simulink library "typhoonPatterns"  (R2019a)
settings: Solver=VariableStepAuto  StartTime=0.0  StopTime=10.0  RelTol=1e-3
undefined symbols (not defined in the file or in its folder): c_clamp, C_l, c_picoup_mat, c_picoup_seq, cc_berg, crun_sp_ind, cst_sp_ind, f, f_picoup, f_sp_ind, fc, Jm, L, L1, L2, L_l, l_picoup_mat, l_picoup_seq, l_rl, La_DC, lc_berg, Lc_sm, Ld, length_rl, Lf_DC, Llfd_sm, Llkd_sm, Llkq_sm, Llr1_ind, Llr2_ind, Llr_ind, llrm_sp_ind, Lls_ind, Lls_sm, llsa_sp_ind, llsm_sp_ind, Lm, Lmd_sm, Lmq_sm, Lq, n1, n2, nanm_sp_ind, pms, R, R1, R2, r_clamp, R_l, r_picoup_mat, r_picoup_seq, r_rl, Ra_DC, rc_berg, Rf_DC, Rf_sm, Rkd_sm, Rkq_sm, Rm, Rr1_ind ... (+10)
libraries: powerlib x281
(part 3 of 3)

== system typhoonPatterns/RL Section 4PH ==
  RL1 : powerlib/Elements/Series RLC Branch  LConnTagsString=__new0  RConnTagsString=__new0  BranchType=RL  Resistance=R  Inductance=L  SetiL0=off  InitialCurrent=0  Capacitance=1e-6  Setx0=off  InitialVoltage=0  Measurements=None
      settings: SourceProductName=Simscape Electrical
  RL2 : powerlib/Elements/Series RLC Branch  LConnTagsString=__new0  RConnTagsString=__new0  BranchType=RL  Resistance=r_rl*length_rl  Inductance=l_rl*length_rl  SetiL0=off  InitialCurrent=0  Capacitance=1e-6  Setx0=off  InitialVoltage=0  Measurements=None
      settings: SourceProductName=Simscape Electrical
  RL3 : powerlib/Elements/Series RLC Branch  LConnTagsString=__new0  RConnTagsString=__new0  BranchType=RL  Resistance=r_rl*length_rl  Inductance=l_rl*length_rl  SetiL0=off  InitialCurrent=0  Capacitance=1e-6  Setx0=off  InitialVoltage=0  Measurements=None
      settings: SourceProductName=Simscape Electrical
  RL4 : powerlib/Elements/Series RLC Branch  LConnTagsString=__new0  RConnTagsString=__new0  BranchType=RL  Resistance=r_rl*length_rl  Inductance=l_rl*length_rl  SetiL0=off  InitialCurrent=0  Capacitance=1e-6  Setx0=off  InitialVoltage=0  Measurements=None
      settings: SourceProductName=Simscape Electrical
  a_in : PMIOPort  Side=Left
  a_out : PMIOPort  Port=2  Side=Right
  b_in : PMIOPort  Port=3  Side=Left
  b_out : PMIOPort  Port=4  Side=Right
  c_in : PMIOPort  Port=5  Side=Left
  c_out : PMIOPort  Port=6  Side=Right
  d_in : PMIOPort  Port=7  Side=Left
  d_out : PMIOPort  Port=8  Side=Right
  connections:
  RL2/RConn1 -- b_out/RConn1
  a_out/RConn1 -- RL1/RConn1
  a_in/RConn1 -- RL1/LConn1
  RL2/LConn1 -- b_in/RConn1
  RL3/LConn1 -- c_in/RConn1
  RL3/RConn1 -- c_out/RConn1
  RL4/RConn1 -- d_out/RConn1
  RL4/LConn1 -- d_in/RConn1

== system typhoonPatterns/RL Section 5PH ==
  RL1 : powerlib/Elements/Series RLC Branch  LConnTagsString=__new0  RConnTagsString=__new0  BranchType=RL  Resistance=R  Inductance=L  SetiL0=off  InitialCurrent=0  Capacitance=1e-6  Setx0=off  InitialVoltage=0  Measurements=None
      settings: SourceProductName=Simscape Electrical
  RL{2..5} (4 alike) : powerlib/Elements/Series RLC Branch  LConnTagsString=__new0  RConnTagsString=__new0  BranchType=RL  Resistance=r_rl*length_rl  Inductance=l_rl*length_rl  SetiL0=off  InitialCurrent=0  Capacitance=1e-6  Setx0=off  InitialVoltage=0  Measurements=None
      settings: SourceProductName=Simscape Electrical
  a_in : PMIOPort  Side=Left
  a_out : PMIOPort  Port=2  Side=Right
  b_in : PMIOPort  Port=3  Side=Left
  b_out : PMIOPort  Port=4  Side=Right
  c_in : PMIOPort  Port=5  Side=Left
  c_out : PMIOPort  Port=6  Side=Right
  d_in : PMIOPort  Port=7  Side=Left
  d_out : PMIOPort  Port=8  Side=Right
  e_in : PMIOPort  Port=9  Side=Left
  e_out : PMIOPort  Port=10  Side=Right
  connections:
  RL4/LConn1 -- d_in/RConn1
  RL4/RConn1 -- d_out/RConn1
  RL3/RConn1 -- c_out/RConn1
  RL3/LConn1 -- c_in/RConn1
  RL2/LConn1 -- b_in/RConn1
  a_in/RConn1 -- RL1/LConn1
  a_out/RConn1 -- RL1/RConn1
  RL2/RConn1 -- b_out/RConn1
  RL5/RConn1 -- e_out/RConn1
  RL5/LConn1 -- e_in/RConn1

== system typhoonPatterns/SP 2W Transformer ==
  T1 : powerlib/Elements/Multi-Winding Transformer  LeftWindings=1  RightWindings=1  TappedWindings=no taps  NumberOfTaps=2  SetSaturation=off  Hysteresis=off  DataFile='hysteresis.mat'  Measurements=None  UNITS=SI  NominalPower=[1, 1]  NominalVoltages=[1,1]  WindingResistances=[1 1]  WindingInductances=[1,1]  Rm=1  Lm=1  Saturation=[0 0;0.0033941 0.27009;1.4142 0.34212]  BreakLoop=off  DiscreteSolver=Trapezoidal iterative  DataType=on  InitialFlux=0  TransfoNumber=1
      settings: AttributesFormatString=%<MaskType>  SourceProductName=Simscape Electrical  SourceProductBaseCode=PS
  prm_1 : PMIOPort  Side=Left
  prm_2 : PMIOPort  Port=2  Side=Left
  sec_1 : PMIOPort  Port=3  Side=Right
  sec_2 : PMIOPort  Port=4  Side=Right
  connections:
  sec_1/RConn1 -- T1/RConn1
  sec_2/RConn1 -- T1/RConn2
  prm_1/RConn1 -- T1/LConn1
  prm_2/RConn1 -- T1/LConn2

== system typhoonPatterns/SP 3W Transformer ==
  T1 : powerlib/Elements/Multi-Winding Transformer  LeftWindings=1  RightWindings=2  TappedWindings=no taps  NumberOfTaps=2  SetSaturation=off  Hysteresis=off  DataFile='hysteresis.mat'  Measurements=None  UNITS=SI  NominalPower=[1,1]  NominalVoltages=[1,1,1]  WindingResistances=[1 1 1]  WindingInductances=[1,1,1,1]  Rm=1  Lm=1  Saturation=[0 0;0.0033941 0.27009;1.4142 0.34212]  BreakLoop=off  DiscreteSolver=Trapezoidal iterative  DataType=on  InitialFlux=0  TransfoNumber=1
      settings: AttributesFormatString=%<MaskType>  SourceProductName=Simscape Electrical  SourceProductBaseCode=PS
  prm_1 : PMIOPort  Side=Left
  prm_2 : PMIOPort  Port=2  Side=Left
  sec_1 : PMIOPort  Port=3  Side=Right
  sec_2 : PMIOPort  Port=4  Side=Right
  sec_3 : PMIOPort  Port=5  Side=Right
  sec_4 : PMIOPort  Port=6  Side=Right
  connections:
  sec_2/RConn1 -- T1/RConn2
  T1/LConn2 -- prm_2/RConn1
  T1/RConn1 -- sec_1/RConn1
  T1/LConn1 -- prm_1/RConn1
  T1/RConn3 -- sec_3/RConn1
  T1/RConn4 -- sec_4/RConn1

== system typhoonPatterns/SP 4W Transformer ==
  T1 : powerlib/Elements/Multi-Winding Transformer  LeftWindings=1  RightWindings=3  TappedWindings=no taps  NumberOfTaps=2  SetSaturation=off  Hysteresis=off  DataFile='hysteresis.mat'  Measurements=None  UNITS=SI  NominalPower=[1, 1]  NominalVoltages=[1,1,1,1]  WindingResistances=[1 1 1 1]  WindingInductances=[1 1 1 1]  Rm=1  Lm=1  Saturation=[0 0;0.0048 0.060792;2 0.077004]  BreakLoop=off  DiscreteSolver=Trapezoidal iterative  DataType=on  InitialFlux=0  TransfoNumber=1
      settings: AttributesFormatString=%<MaskType>  SourceProductName=Simscape Electrical  SourceProductBaseCode=PS
  prm_1 : PMIOPort  Side=Left
  prm_2 : PMIOPort  Port=2  Side=Left
  sec_1 : PMIOPort  Port=3  Side=Right
  sec_2 : PMIOPort  Port=4  Side=Right
  sec_3 : PMIOPort  Port=5  Side=Right
  sec_4 : PMIOPort  Port=6  Side=Right
  sec_5 : PMIOPort  Port=7  Side=Right
  sec_6 : PMIOPort  Port=8  Side=Right
  connections:
  T1/RConn4 -- sec_4/RConn1
  T1/RConn3 -- sec_3/RConn1
  T1/LConn1 -- prm_1/RConn1
  T1/RConn1 -- sec_1/RConn1
  T1/LConn2 -- prm_2/RConn1
  sec_2/RConn1 -- T1/RConn2
  T1/RConn5 -- sec_5/RConn1
  T1/RConn6 -- sec_6/RConn1

== system typhoonPatterns/SP CC ==
  a_in : PMIOPort  Side=Left
  b_in : PMIOPort  Port=2  Side=Left
  a_out : PMIOPort  Port=3  Side=Right
  b_out : PMIOPort  Port=4  Side=Right
  connections:
  a_in/RConn1 -- a_out/RConn1
  b_in/RConn1 -- b_out/RConn1

== system typhoonPatterns/SP Induction Machine ==
  mech : Inport
  Bus Selector : BusSelector  OutputSignals=Mechanical.Rotor speed (rad/s or pu),Mechanical.Electromagnetic torque Te (N*m or pu)
  SP Asynchronous Machine1 : powerlib/Machines/Single Phase Asynchronous Machine  MechanicalLoad=Torque Tm  UNITS=SI  MachineType=Split Phase  MeasurementBus=off  NominalParameters="[0  0  f_sp_ind]"  MainWindingStator="[rsm_sp_ind  llsm_sp_ind]"  MainWindingRotor="[rrm_sp_ind  llrm_sp_ind]"  MutualInductance=lmm_sp_ind  AuxiliaryWinding="[rsa_sp_ind  llsa_sp_ind]"  Mechanical="[Jm  fc pms nanm_sp_ind]"  CapacitorStart="[rst_sp_ind  cst_sp_ind]"  CapacitorRun=[rrun_sp_ind crun_sp_ind]  DisconnectionSpeed=w_disc  InitialSpeed=0  DataType=SI  TsPowergui=0  TsBlock=-1
      settings: SourceProductName=Simscape Electrical  SourceProductBaseCode=PS
  input_rate : RateTransition
  rate_trans : RateTransition  OutPortSampleTime=execution_rate
  A : PMIOPort  Side=Left
  B : PMIOPort  Port=2  Side=Left
  meas : Outport
  w : Outport  Port=2
  T : Outport  Port=3
  wires:
  mech/1 -> input_rate/1
  Bus Selector/1 -> w/1  "<Rotor speed (rad/s or pu)>"
  Bus Selector/2 -> T/1  "<Electromagnetic torque Te (N*m or pu)>"
  SP Asynchronous Machine1/1 -> rate_trans/1, meas/1
  rate_trans/1 -> Bus Selector/1
  input_rate/1 -> SP Asynchronous Machine1/1
  connections:
  SP Asynchronous Machine1/LConn1 -- A/RConn1
  SP Asynchronous Machine1/LConn2 -- B/RConn1

== system typhoonPatterns/SPDT Contactor ==
  control : Inport
  Sa_1 : powerlib/Power Electronics/Ideal Switch  Ron=r_on  Lon=0  IC=s0  Rs=r_s  Cs=c_s  Measurements=on
      settings: SourceProductName=Simscape Electrical
  Sa_2 : powerlib/Power Electronics/Ideal Switch  Ron=r_on  Lon=0  IC=s0  Rs=r_s  Cs=c_s  Measurements=on
      settings: SourceProductName=Simscape Electrical
  inv1 : Logic  Commented=through  Operator=NOT  AllPortsSameDT=off  OutDataTypeStr=boolean
  inv2 : Logic  Operator=NOT  AllPortsSameDT=off  OutDataTypeStr=boolean
  A : PMIOPort  Side=Left
  B : PMIOPort  Port=2  Side=Left
  C : PMIOPort  Port=3  Side=Right
  wires:
  inv1/1 -> inv2/1, [S_1]
  control/1 -> inv1/1
  inv2/1 -> [S_2]
  [S_1] -> Sa_1/1
  [S_2] -> Sa_2/1
  connections:
  A/RConn1 -- Sa_1/LConn1
  B/RConn1 -- Sa_2/LConn1
  C/RConn1 -- Sa_1/RConn1 -- Sa_2/RConn1

== system typhoonPatterns/SPST Contactor ==
  control : Inport
  Sa : powerlib/Power Electronics/Ideal Switch  Ron=r_on  Lon=0  IC=s0  Rs=r_s  Cs=c_s  Measurements=on
      settings: SourceProductName=Simscape Electrical
  inv1 : Logic  Commented=through  Operator=NOT  AllPortsSameDT=off  OutDataTypeStr=boolean
  A : PMIOPort  Side=Left
  B : PMIOPort  Port=2  Side=Right
  wires:
  control/1 -> inv1/1
  inv1/1 -> Sa/1
  connections:
  B/RConn1 -- Sa/RConn1
  A/RConn1 -- Sa/LConn1

== system typhoonPatterns/Symmetrical Boost ==
  gates : Inport
  Boost Converter : powerlib/Power Electronics/Boost Converter  ModelType=Switching devices  Ron=r_on  Rs=r_s  Cs=c_s  Vforward=[0, 0]  Ron_Diode=1e-3  Rs_Diode=1e6  Cs_Diode=inf  Vf_Diode=1e-3  Rs_CurrentSource=inf
      settings: SourceProductName=Simscape Electrical  SourceProductBaseCode=PS
  Buck Converter : powerlib/Power Electronics/Buck Converter  ModelType=Switching devices  Ron=r_on  Rs=r_s  Cs=c_s  Vforward=[0, 0]  Ron_Diode=1e-3  Rs_Diode=1e6  Cs_Diode=inf  Vf_Diode=1e-3  Rs_CurrentSource=inf
      settings: SourceProductName=Simscape Electrical  SourceProductBaseCode=PS
  Demux : Demux  Outputs=2
  inv1 : Logic  Commented=through  Operator=NOT  AllPortsSameDT=off  OutDataTypeStr=boolean
  inv2 : Logic  Commented=through  Operator=NOT  AllPortsSameDT=off  OutDataTypeStr=boolean
  In+ : PMIOPort  Side=Left
  Out+ : PMIOPort  Port=2  Side=Right
  Out- : PMIOPort  Port=3  Side=Right
  In- : PMIOPort  Port=4  Side=Left
  wires:
  [S1] -> Boost Converter/1
  [S2] -> Buck Converter/1
  gates/1 -> Demux/1
  Demux/2 -> inv2/1
  Demux/1 -> inv1/1
  inv1/1 -> [S1]
  inv2/1 -> [S2]
  connections:
  In+/RConn1 -- Boost Converter/RConn1
  Buck Converter/RConn1 -- Boost Converter/RConn2
  Out+/RConn1 -- Boost Converter/LConn1
  Out-/RConn1 -- Buck Converter/RConn2
  In-/RConn1 -- Buck Converter/LConn1

== system typhoonPatterns/Synchronous Machine ==
  mech : Inport
  Bus Selector : BusSelector  OutputSignals="Mechanical.Rotor speed  wm (rad/s),Mechanical.Electromagnetic torque  Te (N*m),Mechanical.Rotor angle deviation  d_theta (rad)"
  Synchronous Machine1 : powerlib/Machines/Synchronous Machine SI Fundamental  PresetModel=No  MechanicalLoad=Mechanical power Pm  ShowDetailedParameters=on  RotorType=Salient-pole  Units=SI fundamental parameters  MeasurementBus=off  NominalParameters="[ 1  1   60   1 ]"  Stator="[Rs_sm  Lls_sm  Lmd_sm  Lmq_sm Lc_sm]"  Field="[ Rf_sm  Llfd_sm ]"  Dampers2=[ 0.0664, 1.387e-3, 0.0292, 6.896e-4, 7.907e-3, 2.477e-3]  Dampers1="[ Rkd_sm  Llkd_sm  Rkq_sm  Llkq_sm]"  Mechanical=[ Jm fc pms ]  PolePairs=pms  InitialConditions="[ 0  0  0  0  0  0  0  0  0 ]"  SetSaturation=off  Saturation=[695.64,774.7,917.5,1001.6,1082.2,1175.9,1293.6,1430.2,1583.7;9660,10623,12243,13063,13757,14437,15180,15890,16567]  DisplayVfd=off  LoadFlowParameters=[1,0,0,0,0]  TsPowergui=0  TsBlock=-1  IterativeModel=Trapezoidal non iterative  IterativeDiscreteModel=Trapezoidal non iterative  BusType=PV  Pref=0  Qref=0  Qmin=-inf  Qmax=inf  PLF=0  QLF=0
      settings: SourceProductName=Simscape Electrical  SourceProductBaseCode=PS
  Vf : powerlib/Measurements/Voltage Measurement  PhasorSimulation=off  OutputType=Complex  PSBequivalent=0
      settings: SourceProductName=Simscape Electrical
  input_rate : RateTransition
  rate_trans : RateTransition  OutPortSampleTime=execution_rate
  A : PMIOPort  Side=Left
  B : PMIOPort  Port=2  Side=Left
  C : PMIOPort  Port=3  Side=Left
  R+ : PMIOPort  Port=4  Side=Right
  R- : PMIOPort  Port=5  Side=Right
  meas : Outport
  w : Outport  Port=2
  T : Outport  Port=3
  theta : Outport  Port=4
  wires:
  input_rate/1 -> Synchronous Machine1/1
  rate_trans/1 -> Bus Selector/1
  Bus Selector/3 -> theta/1  "<Rotor angle deviation  d_theta (rad)>"
  Bus Selector/1 -> w/1  "<Rotor speed  wm (rad/s)>"
  Bus Selector/2 -> T/1  "<Electromagnetic torque  Te (N*m)>"
  Synchronous Machine1/1 -> meas/1, rate_trans/1
  mech/1 -> input_rate/1
  Vf/1 -> Synchronous Machine1/2
  connections:
  Synchronous Machine1/RConn3 -- C/RConn1
  Synchronous Machine1/RConn2 -- B/RConn1
  Synchronous Machine1/RConn1 -- A/RConn1
  Vf/LConn1 -- R+/RConn1
  Vf/LConn2 -- R-/RConn1

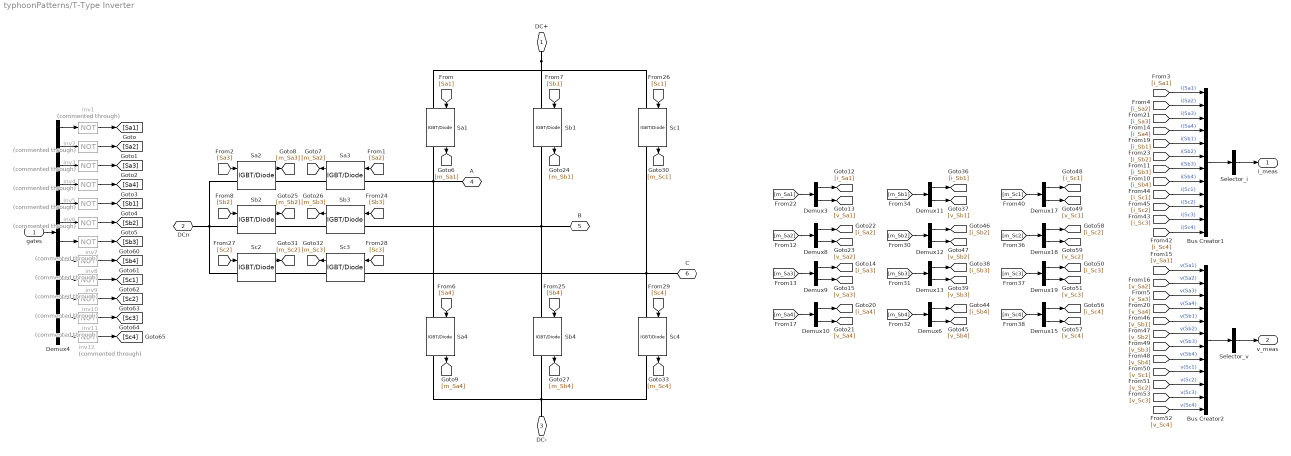
== system typhoonPatterns/T-Type Inverter ==
  gates : Inport
  Bus Creator1 : BusCreator  Inputs=12
  Bus Creator2 : BusCreator  Inputs=12
  Demux{3,6,8..13,15,17..19} (12 alike) : Demux  Outputs=2
  Demux4 : Demux  Outputs=12
  Sa{1..4} (4 alike) : powerlib/Power Electronics/IGBT//Diode  Ron=r_on  Rs=r_s  Cs=c_s  Measurements=on
      settings: SourceProductName=Simscape Electrical
  Sb{1..4} (4 alike) : powerlib/Power Electronics/IGBT//Diode  Ron=r_on  Rs=r_s  Cs=c_s  Measurements=on
      settings: SourceProductName=Simscape Electrical
  Sc{1..4} (4 alike) : powerlib/Power Electronics/IGBT//Diode  Ron=r_on  Rs=r_s  Cs=c_s  Measurements=on
      settings: SourceProductName=Simscape Electrical
  Selector_i : BusSelector  OutputSignals=i(Sa1)  OutputAsBus=on
  Selector_v : BusSelector  OutputSignals=v(Sa1)  OutputAsBus=on
  inv{1..12} (12 alike) : Logic  Commented=through  Operator=NOT  AllPortsSameDT=off  OutDataTypeStr=boolean
  DC+ : PMIOPort  Side=Left
  DCn : PMIOPort  Port=2  Side=Left
  DC- : PMIOPort  Port=3  Side=Left
  A : PMIOPort  Port=4  Side=Right
  B : PMIOPort  Port=5  Side=Right
  C : PMIOPort  Port=6  Side=Right
  i_meas : Outport
  v_meas : Outport  Port=2
  wires:
  [v_Sc1] -> Bus Creator2/9  "v(Sc1)"
  [v_Sc2] -> Bus Creator2/10  "v(Sc2)"
  [v_Sc3] -> Bus Creator2/11  "v(Sc3)"
  [v_Sc4] -> Bus Creator2/12  "v(Sc4)"
  [v_Sb1] -> Bus Creator2/5  "v(Sb1)"
  [v_Sb2] -> Bus Creator2/6  "v(Sb2)"
  [v_Sb3] -> Bus Creator2/7  "v(Sb3)"
  [v_Sb4] -> Bus Creator2/8  "v(Sb4)"
  [i_Sc2] -> Bus Creator1/10  "i(Sc2)"
  [i_Sc3] -> Bus Creator1/11  "i(Sc3)"
  [i_Sc4] -> Bus Creator1/12  "i(Sc4)"
  [i_Sc1] -> Bus Creator1/9  "i(Sc1)"
  [i_Sb2] -> Bus Creator1/6  "i(Sb2)"
  [i_Sb3] -> Bus Creator1/7  "i(Sb3)"
  [i_Sb4] -> Bus Creator1/8  "i(Sb4)"
  [i_Sb1] -> Bus Creator1/5  "i(Sb1)"
  Demux17/1 -> [i_Sc1]
  Demux15/1 -> [i_Sc4]
  [m_Sc2] -> Demux18/1
  [m_Sc1] -> Demux17/1
  Demux19/1 -> [i_Sc3]
  Demux19/2 -> [v_Sc3]
  Demux17/2 -> [v_Sc1]
  Demux18/2 -> [v_Sc2]
  [m_Sc4] -> Demux15/1
  Demux15/2 -> [v_Sc4]
  Demux18/1 -> [i_Sc2]
  [m_Sc3] -> Demux19/1
  Demux11/1 -> [i_Sb1]
  Demux6/1 -> [i_Sb4]
  [m_Sb2] -> Demux12/1
  [m_Sb1] -> Demux11/1
  Demux13/1 -> [i_Sb3]
  Demux13/2 -> [v_Sb3]
  Demux11/2 -> [v_Sb1]
  Demux12/2 -> [v_Sb2]
  [m_Sb4] -> Demux6/1
  Demux6/2 -> [v_Sb4]
  Demux12/1 -> [i_Sb2]
  [m_Sb3] -> Demux13/1
  [Sc2] -> Sc2/1
  Sc1/1 -> [m_Sc1]
  Sc4/1 -> [m_Sc4]
  Sc2/1 -> [m_Sc2]
  [Sc1] -> Sc1/1
  Sc3/1 -> [m_Sc3]
  [Sc3] -> Sc3/1
  [Sc4] -> Sc4/1
  [Sb2] -> Sb2/1
  Sb1/1 -> [m_Sb1]
  Sb4/1 -> [m_Sb4]
  Sb2/1 -> [m_Sb2]
  [Sb1] -> Sb1/1
  Sb3/1 -> [m_Sb3]
  [Sb3] -> Sb3/1
  [Sb4] -> Sb4/1
  [Sa2] -> Sa3/1
  Sa1/1 -> [m_Sa1]
  Sa4/1 -> [m_Sa4]
  Sa3/1 -> [m_Sa2]
  [Sa1] -> Sa1/1
  Sa2/1 -> [m_Sa3]
  [Sa3] -> Sa2/1
  [Sa4] -> Sa4/1
  Selector_v/1 -> v_meas/1
  Demux3/1 -> [i_Sa1]
  [v_Sa4] -> Bus Creator2/4  "v(Sa4)"
  [v_Sa3] -> Bus Creator2/3  "v(Sa3)"
  [i_Sa4] -> Bus Creator1/4  "i(Sa4)"
  Demux3/2 -> [v_Sa1]
  Demux8/1 -> [i_Sa2]
  Bus Creator2/1 -> Selector_v/1
  [i_Sa1] -> Bus Creator1/1  "i(Sa1)"
  Demux9/2 -> [v_Sa3]
  Demux9/1 -> [i_Sa3]
  [v_Sa1] -> Bus Creator2/1  "v(Sa1)"
  Demux8/2 -> [v_Sa2]
  [i_Sa3] -> Bus Creator1/3  "i(Sa3)"
  Demux10/2 -> [v_Sa4]
  [m_Sa2] -> Demux8/1
  [m_Sa3] -> Demux9/1
  [m_Sa4] -> Demux10/1
  Demux10/1 -> [i_Sa4]
  Bus Creator1/1 -> Selector_i/1
  [v_Sa2] -> Bus Creator2/2  "v(Sa2)"
  Selector_i/1 -> i_meas/1
  [m_Sa1] -> Demux3/1
  [i_Sa2] -> Bus Creator1/2  "i(Sa2)"
  inv10/1 -> [Sc2]
  Demux4/11 -> inv11/1
  Demux4/12 -> inv12/1
  Demux4/7 -> inv7/1
  Demux4/8 -> inv8/1
  Demux4/9 -> inv9/1
  inv7/1 -> [Sb3]
  Demux4/10 -> inv10/1
  inv12/1 -> [Sc4]
  inv8/1 -> [Sb4]
  inv6/1 -> [Sb2]
  Demux4/6 -> inv6/1
  inv1/1 -> [Sa1]
  inv2/1 -> [Sa2]
  gates/1 -> Demux4/1
  Demux4/4 -> inv4/1
  Demux4/2 -> inv2/1
  Demux4/3 -> inv3/1
  Demux4/5 -> inv5/1
  inv4/1 -> [Sa4]
  Demux4/1 -> inv1/1
  inv9/1 -> [Sc1]
  inv5/1 -> [Sb1]
  inv11/1 -> [Sc3]
  inv3/1 -> [Sa3]
  connections:
  Sc4/RConn1 -- Sb4/RConn1 -- DC-/RConn1 -- Sa4/RConn1
  DC+/RConn1 -- Sc1/LConn1 -- Sb1/LConn1 -- Sa1/LConn1
  Sa2/RConn1 -- Sa3/RConn1
  Sb2/RConn1 -- Sb3/RConn1
  Sc2/RConn1 -- Sc3/RConn1
  Sa4/LConn1 -- A/RConn1 -- Sa3/LConn1 -- Sa1/RConn1
  Sb4/LConn1 -- Sb1/RConn1 -- B/RConn1 -- Sb3/LConn1
  Sc4/LConn1 -- Sc1/RConn1 -- C/RConn1 -- Sc3/LConn1
  Sa2/LConn1 -- DCn/RConn1 -- Sb2/LConn1 -- Sc2/LConn1

== system typhoonPatterns/TP 2W Transformer ==
  T1 : powerlib/Elements/Three-Phase Transformer (Two Windings)  Winding1Connection=Yg  Winding2Connection=Yg  CoreType=Three single-phase transformers  SetSaturation=off  Hysteresis=off  DataFile='hysteresis'  SetInitialFlux=off  Measurements=None  UNITS=SI  NominalPower=[1, 1]  Winding1=[1 1 1]  Winding2=[1 1 1]  Rm=1  Lm=1  L0=0.079577  Saturation=[0 0;0.0019596 0.15594;0.8165 0.19752]  InitialFluxes=[0.10396 -0.10396 0.090965]  BreakLoop=off  DiscreteSolver=Trapezoidal iterative  DataType=on  TransfoNumber=1
      settings: AttributesFormatString=%<MaskType>  SourceProductName=Simscape Electrical
  prm_1 : PMIOPort  Side=Left
  prm_2 : PMIOPort  Port=2  Side=Left
  prm_3 : PMIOPort  Port=3  Side=Left
  sec_1 : PMIOPort  Port=4  Side=Right
  sec_2 : PMIOPort  Port=5  Side=Right
  sec_3 : PMIOPort  Port=6  Side=Right
  connections:
  T1/LConn2 -- prm_2/RConn1
  T1/LConn1 -- prm_1/RConn1
  T1/LConn3 -- prm_3/RConn1
  sec_1/RConn1 -- T1/RConn1
  sec_2/RConn1 -- T1/RConn2
  sec_3/RConn1 -- T1/RConn3

== system typhoonPatterns/TP 3W Transformer ==
  T1 : powerlib/Elements/Three-Phase Transformer (Three Windings)  Winding1Connection=Y  Winding2Connection=Yg  Winding3Connection=Yg  CoreType=Three single-phase transformers  SetSaturation=off  Hysteresis=off  DataFile='hysteresis'  SetInitialFlux=off  Measurements=None  UNITS=SI  NominalPower=[1 , 1]  Winding1=[1 1 1]  Winding2=[1 1 1]  Winding3=[1 1 1]  Rm=1  Lm=1  L0=0.5  Saturation=[0 0;0.0019596 0.15594;0.8165 0.19752]  InitialFluxes=[0.10396 -0.10396 0.090965]  BreakLoop=off  DiscreteSolver=Trapezoidal iterative  DataType=on  TransfoNumber=1
      settings: AttributesFormatString=%<MaskType>  SourceProductName=Simscape Electrical  SourceProductBaseCode=PS
  prm_1 : PMIOPort  Side=Left
  prm_2 : PMIOPort  Port=2  Side=Left
  prm_3 : PMIOPort  Port=3  Side=Left
  sec_1 : PMIOPort  Port=4  Side=Right
  sec_2 : PMIOPort  Port=5  Side=Right
  sec_3 : PMIOPort  Port=6  Side=Right
  sec_4 : PMIOPort  Port=7  Side=Right
  sec_5 : PMIOPort  Port=8  Side=Right
  sec_6 : PMIOPort  Port=9  Side=Right
  connections:
  T1/RConn3 -- sec_3/RConn1
  T1/RConn2 -- sec_2/RConn1
  T1/RConn1 -- sec_1/RConn1
  T1/LConn3 -- prm_3/RConn1
  T1/LConn1 -- prm_1/RConn1
  T1/LConn2 -- prm_2/RConn1
  T1/RConn6 -- sec_6/RConn1
  T1/RConn5 -- sec_5/RConn1
  T1/RConn4 -- sec_4/RConn1

== system typhoonPatterns/TP CC ==
  a_in : PMIOPort  Side=Left
  b_in : PMIOPort  Port=2  Side=Left
  a_out : PMIOPort  Port=3  Side=Right
  b_out : PMIOPort  Port=4  Side=Right
  c_in : PMIOPort  Port=5  Side=Left
  c_out : PMIOPort  Port=6  Side=Right
  connections:
  a_in/RConn1 -- a_out/RConn1
  b_in/RConn1 -- b_out/RConn1
  c_in/RConn1 -- c_out/RConn1

== system typhoonPatterns/TPDT Contactor ==
  control : Inport
  Sa_1 : powerlib/Power Electronics/Ideal Switch  Ron=r_on  Lon=0  IC=s0  Rs=r_s  Cs=c_s  Measurements=on
      settings: SourceProductName=Simscape Electrical
  Sa_2 : powerlib/Power Electronics/Ideal Switch  Ron=r_on  Lon=0  IC=s0  Rs=r_s  Cs=c_s  Measurements=on
      settings: SourceProductName=Simscape Electrical
  Sb_1 : powerlib/Power Electronics/Ideal Switch  Ron=r_on  Lon=0  IC=s0  Rs=r_s  Cs=c_s  Measurements=on
      settings: SourceProductName=Simscape Electrical
  Sb_2 : powerlib/Power Electronics/Ideal Switch  Ron=r_on  Lon=0  IC=s0  Rs=r_s  Cs=c_s  Measurements=on
      settings: SourceProductName=Simscape Electrical
  Sc_1 : powerlib/Power Electronics/Ideal Switch  Ron=r_on  Lon=0  IC=s0  Rs=r_s  Cs=c_s  Measurements=on
      settings: SourceProductName=Simscape Electrical
  Sc_2 : powerlib/Power Electronics/Ideal Switch  Ron=r_on  Lon=0  IC=s0  Rs=r_s  Cs=c_s  Measurements=on
      settings: SourceProductName=Simscape Electrical
  inv1 : Logic  Commented=through  Operator=NOT  AllPortsSameDT=off  OutDataTypeStr=boolean
  inv2 : Logic  Operator=NOT  AllPortsSameDT=off  OutDataTypeStr=boolean
  A1 : PMIOPort  Side=Left
  B1 : PMIOPort  Port=2  Side=Left
  C1 : PMIOPort  Port=3  Side=Right
  A2 : PMIOPort  Port=4  Side=Left
  B2 : PMIOPort  Port=5  Side=Left
  C2 : PMIOPort  Port=6  Side=Right
  A3 : PMIOPort  Port=7  Side=Left
  B3 : PMIOPort  Port=8  Side=Left
  C3 : PMIOPort  Port=9  Side=Right
  wires:
  [S_1] -> Sb_1/1
  [S_2] -> Sb_2/1
  inv1/1 -> inv2/1, [S_1]
  control/1 -> inv1/1
  inv2/1 -> [S_2]
  [S_1] -> Sa_1/1
  [S_2] -> Sa_2/1
  [S_2] -> Sc_2/1
  [S_1] -> Sc_1/1
  connections:
  B2/RConn1 -- Sb_2/LConn1
  A2/RConn1 -- Sb_1/LConn1
  Sb_1/RConn1 -- Sb_2/RConn1 -- C2/RConn1
  A1/RConn1 -- Sa_1/LConn1
  B1/RConn1 -- Sa_2/LConn1
  Sa_2/RConn1 -- C1/RConn1 -- Sa_1/RConn1
  C3/RConn1 -- Sc_1/RConn1 -- Sc_2/RConn1
  B3/RConn1 -- Sc_2/LConn1
  A3/RConn1 -- Sc_1/LConn1

== system typhoonPatterns/TPST Contactor ==
  control : Inport
  Sa : powerlib/Power Electronics/Ideal Switch  Ron=r_on  Lon=0  IC=s0  Rs=r_s  Cs=c_s  Measurements=on
      settings: SourceProductName=Simscape Electrical
  Sb : powerlib/Power Electronics/Ideal Switch  Ron=r_on  Lon=0  IC=s0  Rs=r_s  Cs=c_s  Measurements=on
      settings: SourceProductName=Simscape Electrical
  Sc : powerlib/Power Electronics/Ideal Switch  Ron=r_on  Lon=0  IC=s0  Rs=r_s  Cs=c_s  Measurements=on
      settings: SourceProductName=Simscape Electrical
  inv1 : Logic  Commented=through  Operator=NOT  AllPortsSameDT=off  OutDataTypeStr=boolean
  A1 : PMIOPort  Side=Left
  B1 : PMIOPort  Port=2  Side=Right
  A2 : PMIOPort  Port=3  Side=Left
  B2 : PMIOPort  Port=4  Side=Right
  A3 : PMIOPort  Port=5  Side=Left
  B3 : PMIOPort  Port=6  Side=Right
  wires:
  inv1/1 -> [S]
  [S] -> Sb/1
  control/1 -> inv1/1
  [S] -> Sa/1
  [S] -> Sc/1
  connections:
  B2/RConn1 -- Sb/RConn1
  A1/RConn1 -- Sa/LConn1
  A2/RConn1 -- Sb/LConn1
  B1/RConn1 -- Sa/RConn1
  A3/RConn1 -- Sc/LConn1
  B3/RConn1 -- Sc/RConn1

== system typhoonPatterns/Thyristor Rectifier (1-Phase) ==
  gates : Inport
  Bus Creator : BusCreator  Inputs=4
  Bus Creator1 : BusCreator  Inputs=4
  Demux{1..3,5} (4 alike) : Demux  Outputs=2
  Demux4 : Demux
  Selector_i : BusSelector  OutputSignals=i(Sa_top)  OutputAsBus=on
  Selector_v : BusSelector  OutputSignals=v(Sa_top)  OutputAsBus=on
  inv{1..4} (4 alike) : Logic  Commented=through  Operator=NOT  AllPortsSameDT=off  OutDataTypeStr=boolean
  sa_bot : powerlib/Power Electronics/Thyristor  Ron=r_on  Lon=0  Vf=v_f  IC=0  Rs=r_s  Cs=c_s  Measurements=on
      settings: SourceProductName=Simscape Electrical
  sa_top : powerlib/Power Electronics/Thyristor  Ron=r_on  Lon=0  Vf=v_f  IC=0  Rs=r_s  Cs=c_s  Measurements=on
      settings: SourceProductName=Simscape Electrical
  sb_bot : powerlib/Power Electronics/Thyristor  Ron=r_on  Lon=0  Vf=v_f  IC=0  Rs=r_s  Cs=c_s  Measurements=on
      settings: SourceProductName=Simscape Electrical
  sb_top : powerlib/Power Electronics/Thyristor  Ron=r_on  Lon=0  Vf=v_f  IC=0  Rs=r_s  Cs=c_s  Measurements=on
      settings: SourceProductName=Simscape Electrical
  A : PMIOPort  Side=Left
  B : PMIOPort  Port=2  Side=Left
  DC+ : PMIOPort  Port=3  Side=Right
  DC- : PMIOPort  Port=4  Side=Right
  i_meas : Outport
  v_meas : Outport  Port=2
  wires:
  inv4/1 -> [Sb_bot]
  sb_top/1 -> [m_Sb_top]
  [Sb_top] -> sb_top/1
  sa_bot/1 -> [m_Sa_bot]
  Demux4/4 -> inv4/1
  [Sa_top] -> sa_top/1
  Demux4/2 -> inv2/1
  inv2/1 -> [Sa_bot]
  [Sa_bot] -> sa_bot/1
  sb_bot/1 -> [m_Sb_bot]
  gates/1 -> Demux4/1
  inv3/1 -> [Sb_top]
  sa_top/1 -> [m_Sa_top]
  Demux4/3 -> inv3/1
  inv1/1 -> [Sa_top]
  [Sb_bot] -> sb_bot/1
  Demux4/1 -> inv1/1
  Demux2/2 -> [v_Sa_bot]
  Demux1/2 -> [v_Sa_top]
  [v_Sa_top] -> Bus Creator1/1  "v(Sa_top)"
  [i_Sb_top] -> Bus Creator/3  "i(Sb_top)"
  [i_Sb_bot] -> Bus Creator/4  "i(Sb_bot)"
  Demux5/2 -> [v_Sb_bot]
  Bus Creator1/1 -> Selector_v/1
  Demux3/2 -> [v_Sb_top]
  [v_Sb_bot] -> Bus Creator1/4  "v(Sb_bot)"
  Demux5/1 -> [i_Sb_bot]
  Selector_v/1 -> v_meas/1
  [v_Sb_top] -> Bus Creator1/3  "v(Sb_top)"
  [m_Sb_bot] -> Demux5/1
  [m_Sa_bot] -> Demux2/1
  Demux1/1 -> [i_Sa_top]
  [m_Sa_top] -> Demux1/1
  Bus Creator/1 -> Selector_i/1
  [m_Sb_top] -> Demux3/1
  Demux2/1 -> [i_Sa_bot]
  Selector_i/1 -> i_meas/1
  Demux3/1 -> [i_Sb_top]
  [v_Sa_bot] -> Bus Creator1/2  "v(Sa_bot)"
  [i_Sa_bot] -> Bus Creator/2  "i(Sa_bot)"
  [i_Sa_top] -> Bus Creator/1  "i(Sa_top)"
  connections:
  sa_top/RConn1 -- DC+/RConn1 -- sb_top/RConn1
  sa_bot/LConn1 -- DC-/RConn1 -- sb_bot/LConn1
  sa_bot/RConn1 -- sa_top/LConn1 -- A/RConn1
  sb_bot/RConn1 -- sb_top/LConn1 -- B/RConn1

== system typhoonPatterns/Thyristor Rectifier (3-Phase) ==
  gates : Inport
  Bus Creator1 : BusCreator  Inputs=6
  Bus Creator2 : BusCreator  Inputs=6
  Demux{1..3,8..10} (6 alike) : Demux  Outputs=2
  Demux4 : Demux  Outputs=6
  Selector_i : BusSelector  OutputSignals=i(Sa_top)  OutputAsBus=on
  Selector_v : BusSelector  OutputSignals=v(Sa_top)  OutputAsBus=on
  inv{1..6} (6 alike) : Logic  Commented=through  Operator=NOT  AllPortsSameDT=off  OutDataTypeStr=boolean
  sa_bot : powerlib/Power Electronics/Thyristor  Ron=r_on  Lon=0  Vf=v_f  IC=0  Rs=r_s  Cs=c_s  Measurements=on
      settings: SourceProductName=Simscape Electrical
  sa_top : powerlib/Power Electronics/Thyristor  Ron=r_on  Lon=0  Vf=v_f  IC=0  Rs=r_s  Cs=c_s  Measurements=on
      settings: SourceProductName=Simscape Electrical
  sb_bot : powerlib/Power Electronics/Thyristor  Ron=r_on  Lon=0  Vf=v_f  IC=0  Rs=r_s  Cs=c_s  Measurements=on
      settings: SourceProductName=Simscape Electrical
  sb_top : powerlib/Power Electronics/Thyristor  Ron=r_on  Lon=0  Vf=v_f  IC=0  Rs=r_s  Cs=c_s  Measurements=on
      settings: SourceProductName=Simscape Electrical
  sc_bot : powerlib/Power Electronics/Thyristor  Ron=r_on  Lon=0  Vf=v_f  IC=0  Rs=r_s  Cs=c_s  Measurements=on
      settings: SourceProductName=Simscape Electrical
  sc_top : powerlib/Power Electronics/Thyristor  Ron=r_on  Lon=0  Vf=v_f  IC=0  Rs=r_s  Cs=c_s  Measurements=on
      settings: SourceProductName=Simscape Electrical
  A : PMIOPort  Side=Left
  B : PMIOPort  Port=2  Side=Left
  C : PMIOPort  Port=3  Side=Left
  DC+ : PMIOPort  Port=4  Side=Right
  DC- : PMIOPort  Port=5  Side=Right
  i_meas : Outport
  v_meas : Outport  Port=2
  wires:
  inv2/1 -> [Sa_bot]
  inv3/1 -> [Sb_top]
  Demux4/2 -> inv2/1
  inv1/1 -> [Sa_top]
  Demux4/1 -> inv1/1
  Demux4/3 -> inv3/1
  gates/1 -> Demux4/1
  Demux4/5 -> inv5/1
  inv6/1 -> [Sc_bot]
  Demux4/6 -> inv6/1
  inv4/1 -> [Sb_bot]
  inv5/1 -> [Sc_top]
  Demux4/4 -> inv4/1
  [Sa_top] -> sa_top/1
  [Sa_bot] -> sa_bot/1
  [Sb_top] -> sb_top/1
  [Sb_bot] -> sb_bot/1
  [Sc_top] -> sc_top/1
  [Sc_bot] -> sc_bot/1
  sa_top/1 -> [m_Sa_top]
  sa_bot/1 -> [m_Sa_bot]
  sb_top/1 -> [m_Sb_top]
  sb_bot/1 -> [m_Sb_bot]
  sc_top/1 -> [m_Sc_top]
  sc_bot/1 -> [m_Sc_bot]
  [i_Sa_bot] -> Bus Creator1/2  "i(Sa_bot)"
  Demux9/1 -> [i_Sb_top]
  Demux8/2 -> [v_Sa_bot]
  [m_Sa_top] -> Demux3/1
  Bus Creator1/1 -> Selector_i/1
  Demux9/2 -> [v_Sb_top]
  [m_Sc_bot] -> Demux1/1
  Bus Creator2/1 -> Selector_v/1
  Selector_v/1 -> v_meas/1
  [v_Sa_top] -> Bus Creator2/1  "v(Sa_top)"
  [i_Sb_bot] -> Bus Creator1/4  "i(Sb_bot)"
  [v_Sc_top] -> Bus Creator2/5  "v(Sc_top)"
  Demux2/2 -> [v_Sc_top]
  [i_Sb_top] -> Bus Creator1/3  "i(Sb_top)"
  [v_Sc_bot] -> Bus Creator2/6  "v(Sc_bot)"
  Demux10/2 -> [v_Sb_bot]
  Demux3/1 -> [i_Sa_top]
  [m_Sb_bot] -> Demux10/1
  Demux1/1 -> [i_Sc_bot]
  [i_Sc_top] -> Bus Creator1/5  "i(Sc_top)"
  [i_Sc_bot] -> Bus Creator1/6  "i(Sc_bot)"
  Demux3/2 -> [v_Sa_top]
  [m_Sc_top] -> Demux2/1
  [i_Sa_top] -> Bus Creator1/1  "i(Sa_top)"
  [m_Sb_top] -> Demux9/1
  Selector_i/1 -> i_meas/1
  [m_Sa_bot] -> Demux8/1
  [v_Sa_bot] -> Bus Creator2/2  "v(Sa_bot)"
  Demux1/2 -> [v_Sc_bot]
  Demux10/1 -> [i_Sb_bot]
  Demux2/1 -> [i_Sc_top]
  [v_Sb_top] -> Bus Creator2/3  "v(Sb_top)"
  [v_Sb_bot] -> Bus Creator2/4  "v(Sb_bot)"
  Demux8/1 -> [i_Sa_bot]
  connections:
  sa_bot/RConn1 -- sa_top/LConn1 -- A/RConn1
  sb_bot/RConn1 -- sb_top/LConn1 -- B/RConn1
  sc_bot/RConn1 -- sc_top/LConn1 -- C/RConn1
  sa_top/RConn1 -- DC+/RConn1 -- sc_top/RConn1 -- sb_top/RConn1
  sa_bot/LConn1 -- DC-/RConn1 -- sc_bot/LConn1 -- sb_bot/LConn1

== system typhoonPatterns/VSI (1-Phase) ==
  gates : Inport
  Bus Creator : BusCreator  Inputs=4
  Bus Creator1 : BusCreator  Inputs=4
  Demux{1..3,5} (4 alike) : Demux  Outputs=2
  Demux4 : Demux
  Selector_i : BusSelector  OutputSignals=i(Sa_top)  OutputAsBus=on
  Selector_v : BusSelector  OutputSignals=i(Sa_top)  OutputAsBus=on
  inv{1..4} (4 alike) : Logic  Commented=through  Operator=NOT  AllPortsSameDT=off  OutDataTypeStr=boolean
  sa_bot : powerlib/Power Electronics/IGBT//Diode  Ron=r_on  Rs=r_s  Cs=c_s  Measurements=on
      settings: SourceProductName=Simscape Electrical
  sa_top : powerlib/Power Electronics/IGBT//Diode  Ron=r_on  Rs=r_s  Cs=c_s  Measurements=on
      settings: SourceProductName=Simscape Electrical
  sb_bot : powerlib/Power Electronics/IGBT//Diode  Ron=r_on  Rs=r_s  Cs=c_s  Measurements=on
      settings: SourceProductName=Simscape Electrical
  sb_top : powerlib/Power Electronics/IGBT//Diode  Ron=r_on  Rs=r_s  Cs=c_s  Measurements=on
      settings: SourceProductName=Simscape Electrical
  A : PMIOPort  Side=Right
  B : PMIOPort  Port=2  Side=Right
  DC+ : PMIOPort  Port=3  Side=Left
  DC- : PMIOPort  Port=4  Side=Left
  i_meas : Outport
  v_meas : Outport  Port=2
  wires:
  [i_Sa_top] -> Bus Creator/1  "i(Sa_top)"
  [i_Sa_bot] -> Bus Creator/2  "i(Sa_bot)"
  [v_Sa_bot] -> Bus Creator1/2  "v(Sa_bot)"
  Demux3/1 -> [i_Sb_top]
  Selector_i/1 -> i_meas/1
  Demux2/1 -> [i_Sa_bot]
  [m_Sb_top] -> Demux3/1
  Bus Creator/1 -> Selector_i/1
  [m_Sa_top] -> Demux1/1
  Demux1/1 -> [i_Sa_top]
  [m_Sa_bot] -> Demux2/1
  [m_Sb_bot] -> Demux5/1
  [v_Sb_top] -> Bus Creator1/3  "v(Sb_top)"
  Selector_v/1 -> v_meas/1
  Demux5/1 -> [i_Sb_bot]
  [v_Sb_bot] -> Bus Creator1/4  "v(Sb_bot)"
  Demux3/2 -> [v_Sb_top]
  Bus Creator1/1 -> Selector_v/1
  Demux5/2 -> [v_Sb_bot]
  [i_Sb_bot] -> Bus Creator/4  "i(Sb_bot)"
  [i_Sb_top] -> Bus Creator/3  "i(Sb_top)"
  [v_Sa_top] -> Bus Creator1/1  "v(Sa_top)"
  Demux1/2 -> [v_Sa_top]
  Demux2/2 -> [v_Sa_bot]
  Demux4/1 -> inv1/1
  inv1/1 -> [Sa_top]
  Demux4/3 -> inv3/1
  inv3/1 -> [Sb_top]
  gates/1 -> Demux4/1
  inv2/1 -> [Sa_bot]
  Demux4/2 -> inv2/1
  Demux4/4 -> inv4/1
  inv4/1 -> [Sb_bot]
  sa_top/1 -> [m_Sa_top]
  [Sa_top] -> sa_top/1
  sa_bot/1 -> [m_Sa_bot]
  [Sa_bot] -> sa_bot/1
  sb_bot/1 -> [m_Sb_bot]
  [Sb_bot] -> sb_bot/1
  sb_top/1 -> [m_Sb_top]
  [Sb_top] -> sb_top/1
  connections:
  DC-/RConn1 -- sb_bot/RConn1 -- sa_bot/RConn1
  sa_top/RConn1 -- A/RConn1 -- sa_bot/LConn1
  sb_top/RConn1 -- B/RConn1 -- sb_bot/LConn1
  DC+/RConn1 -- sb_top/LConn1 -- sa_top/LConn1

== system typhoonPatterns/VSI (3-Phase) ==
  gates : Inport
  Bus Creator1 : BusCreator  Inputs=6
  Bus Creator2 : BusCreator  Inputs=6
  Demux{1..3,8..10} (6 alike) : Demux  Outputs=2
  Demux4 : Demux  Outputs=6
  Selector_i : BusSelector  OutputSignals=i(Sa_top)  OutputAsBus=on
  Selector_v : BusSelector  OutputSignals=v(Sa_top)  OutputAsBus=on
  inv{1..6} (6 alike) : Logic  Commented=through  Operator=NOT  AllPortsSameDT=off  OutDataTypeStr=boolean
  sa_bot : powerlib/Power Electronics/IGBT//Diode  Ron=r_on  Rs=r_s  Cs=c_s  Measurements=on
      settings: SourceProductName=Simscape Electrical
  sa_top : powerlib/Power Electronics/IGBT//Diode  Ron=r_on  Rs=r_s  Cs=c_s  Measurements=on
      settings: SourceProductName=Simscape Electrical
  sb_bot : powerlib/Power Electronics/IGBT//Diode  Ron=r_on  Rs=r_s  Cs=c_s  Measurements=on
      settings: SourceProductName=Simscape Electrical
  sb_top : powerlib/Power Electronics/IGBT//Diode  Ron=r_on  Rs=r_s  Cs=c_s  Measurements=on
      settings: SourceProductName=Simscape Electrical
  sc_bot : powerlib/Power Electronics/IGBT//Diode  Ron=r_on  Rs=r_s  Cs=c_s  Measurements=on
      settings: SourceProductName=Simscape Electrical
  sc_top : powerlib/Power Electronics/IGBT//Diode  Ron=r_on  Rs=r_s  Cs=c_s  Measurements=on
      settings: SourceProductName=Simscape Electrical
  A : PMIOPort  Side=Right
  B : PMIOPort  Port=2  Side=Right
  DC+ : PMIOPort  Port=3  Side=Left
  DC- : PMIOPort  Port=4  Side=Left
  C : PMIOPort  Port=5  Side=Right
  i_meas : Outport
  v_meas : Outport  Port=2
  wires:
  inv2/1 -> [Sa_bot]
  inv3/1 -> [Sb_top]
  Demux4/2 -> inv2/1
  inv1/1 -> [Sa_top]
  Demux4/1 -> inv1/1
  Demux4/3 -> inv3/1
  gates/1 -> Demux4/1
  Demux4/5 -> inv5/1
  inv6/1 -> [Sc_bot]
  Demux4/6 -> inv6/1
  inv4/1 -> [Sb_bot]
  inv5/1 -> [Sc_top]
  Demux4/4 -> inv4/1
  sa_top/1 -> [m_Sa_top]
  sb_bot/1 -> [m_Sb_bot]
  [Sb_top] -> sb_top/1
  sa_bot/1 -> [m_Sa_bot]
  sb_top/1 -> [m_Sb_top]
  [Sb_bot] -> sb_bot/1
  [Sa_top] -> sa_top/1
  [Sa_bot] -> sa_bot/1
  sc_top/1 -> [m_Sc_top]
  sc_bot/1 -> [m_Sc_bot]
  [Sc_top] -> sc_top/1
  [Sc_bot] -> sc_bot/1
  [i_Sa_bot] -> Bus Creator1/2  "i(Sa_bot)"
  Demux9/1 -> [i_Sb_top]
  Demux8/2 -> [v_Sa_bot]
  [m_Sa_top] -> Demux3/1
  Bus Creator1/1 -> Selector_i/1
  Demux9/2 -> [v_Sb_top]
  [m_Sc_bot] -> Demux1/1
  Bus Creator2/1 -> Selector_v/1
  Selector_v/1 -> v_meas/1
  [v_Sa_top] -> Bus Creator2/1  "v(Sa_top)"
  [i_Sb_bot] -> Bus Creator1/4  "i(Sb_bot)"
  [v_Sc_top] -> Bus Creator2/5  "v(Sc_top)"
  Demux2/2 -> [v_Sc_top]
  [i_Sb_top] -> Bus Creator1/3  "i(Sb_top)"
  [v_Sc_bot] -> Bus Creator2/6  "v(Sc_bot)"
  Demux10/2 -> [v_Sb_bot]
  Demux3/1 -> [i_Sa_top]
  [m_Sb_bot] -> Demux10/1
  Demux1/1 -> [i_Sc_bot]
  [i_Sc_top] -> Bus Creator1/5  "i(Sc_top)"
  [i_Sc_bot] -> Bus Creator1/6  "i(Sc_bot)"
  Demux3/2 -> [v_Sa_top]
  [m_Sc_top] -> Demux2/1
  [i_Sa_top] -> Bus Creator1/1  "i(Sa_top)"
  [m_Sb_top] -> Demux9/1
  Selector_i/1 -> i_meas/1
  [m_Sa_bot] -> Demux8/1
  [v_Sa_bot] -> Bus Creator2/2  "v(Sa_bot)"
  Demux1/2 -> [v_Sc_bot]
  Demux10/1 -> [i_Sb_bot]
  Demux2/1 -> [i_Sc_top]
  [v_Sb_top] -> Bus Creator2/3  "v(Sb_top)"
  [v_Sb_bot] -> Bus Creator2/4  "v(Sb_bot)"
  Demux8/1 -> [i_Sa_bot]
  connections:
  sa_bot/RConn1 -- sc_bot/RConn1 -- sb_bot/RConn1 -- DC-/RConn1
  sa_bot/LConn1 -- A/RConn1 -- sa_top/RConn1
  sb_bot/LConn1 -- B/RConn1 -- sb_top/RConn1
  sa_top/LConn1 -- sc_top/LConn1 -- sb_top/LConn1 -- DC+/RConn1
  sc_bot/LConn1 -- C/RConn1 -- sc_top/RConn1

== system typhoonPatterns/Vienna Rectifier ==
  gates : Inport
  Bus Creator1 : BusCreator  Inputs=3
  Bus Creator2 : BusCreator  Inputs=3
  D{1..6} (6 alike) : powerlib/Power Electronics/Diode  Ron=r_on  Lon=0  Vf=v_f  IC=0  UseSnubber=0  Rs=r_s  Cs=c_s  Measurements=off
      settings: SourceProductName=Simscape Electrical
  Demux : Demux  Outputs=3
  Demux6 : Demux  Outputs=2
  Demux8 : Demux  Outputs=2
  Demux9 : Demux  Outputs=2
  Diode Bridge : powerlib/Power Electronics/Universal Bridge  Arms=2  SnubberResistance=r_s  SnubberCapacitance=c_s  Device=Diodes  Ron=r_on  Lon=0  ForwardVoltages="[  0  0  ]"  ForwardVoltage=v_f  GTOparameters=[ 10e-6 , 20e-6 ]  IGBTparameters=[ 1e-6 , 2e-6 ]  Measurements=None  Measurements_2=None  converterType=Rectifier
      settings: SourceProductName=Simscape Electrical
  Diode Bridge1 : powerlib/Power Electronics/Universal Bridge  Arms=2  SnubberResistance=r_s  SnubberCapacitance=c_s  Device=Diodes  Ron=r_on  Lon=0  ForwardVoltages="[  0  0  ]"  ForwardVoltage=v_f  GTOparameters=[ 10e-6 , 20e-6 ]  IGBTparameters=[ 1e-6 , 2e-6 ]  Measurements=None  Measurements_2=None  converterType=Rectifier
      settings: SourceProductName=Simscape Electrical
  Diode Bridge2 : powerlib/Power Electronics/Universal Bridge  Arms=2  SnubberResistance=r_s  SnubberCapacitance=c_s  Device=Diodes  Ron=r_on  Lon=0  ForwardVoltages="[  0  0  ]"  ForwardVoltage=v_f  GTOparameters=[ 10e-6 , 20e-6 ]  IGBTparameters=[ 1e-6 , 2e-6 ]  Measurements=None  Measurements_2=None  converterType=Rectifier
      settings: SourceProductName=Simscape Electrical
  S_a : powerlib/Power Electronics/IGBT  Ron=r_on  Lon=0  Vf=v_f  Tf=1e-6  Tt=2e-6  IC=0  Rs=r_s  Cs=c_s  Measurements=on
      settings: SourceProductName=Simscape Electrical
  S_b : powerlib/Power Electronics/IGBT  Ron=r_on  Lon=0  Vf=v_f  Tf=1e-6  Tt=2e-6  IC=0  Rs=r_s  Cs=c_s  Measurements=on
      settings: SourceProductName=Simscape Electrical
  S_c : powerlib/Power Electronics/IGBT  Ron=r_on  Lon=0  Vf=v_f  Tf=1e-6  Tt=2e-6  IC=0  Rs=r_s  Cs=c_s  Measurements=on
      settings: SourceProductName=Simscape Electrical
  Selector_i : BusSelector  OutputSignals=i(Sa)  OutputAsBus=on
  Selector_v : BusSelector  OutputSignals=v(Sa)  OutputAsBus=on
  inv1 : Logic  Commented=through  Operator=NOT  AllPortsSameDT=off  OutDataTypeStr=boolean
  inv2 : Logic  Commented=through  Operator=NOT  AllPortsSameDT=off  OutDataTypeStr=boolean
  inv3 : Logic  Commented=through  Operator=NOT  AllPortsSameDT=off  OutDataTypeStr=boolean
  A : PMIOPort  Side=Left
  B : PMIOPort  Port=2  Side=Left
  C : PMIOPort  Port=3  Side=Left
  DC+ : PMIOPort  Port=4  Side=Right
  DCn : PMIOPort  Port=5  Side=Right
  DC- : PMIOPort  Port=6  Side=Right
  i_meas : Outport
  v_meas : Outport  Port=2
  wires:
  gates/1 -> Demux/1
  Demux/1 -> inv1/1
  Demux/2 -> inv2/1
  Demux/3 -> inv3/1
  [Sa] -> S_a/1
  [Sb] -> S_b/1
  [Sc] -> S_c/1
  inv1/1 -> [Sa]
  inv2/1 -> [Sb]
  inv3/1 -> [Sc]
  S_a/1 -> [m_Sa]
  S_b/1 -> [m_Sb]
  S_c/1 -> [m_Sc]
  [m_Sa] -> Demux6/1
  Demux9/1 -> [i_Sc]
  [i_Sa] -> Bus Creator1/1  "i(Sa)"
  Bus Creator1/1 -> Selector_i/1
  [v_Sb] -> Bus Creator2/2  "v(Sb)"
  Selector_i/1 -> i_meas/1
  Selector_v/1 -> v_meas/1
  Demux8/2 -> [v_Sb]
  Demux6/2 -> [v_Sa]
  [i_Sc] -> Bus Creator1/3  "i(Sc)"
  Demux8/1 -> [i_Sb]
  [v_Sc] -> Bus Creator2/3  "v(Sc)"
  Bus Creator2/1 -> Selector_v/1
  [i_Sb] -> Bus Creator1/2  "i(Sb)"
  Demux6/1 -> [i_Sa]
  [m_Sc] -> Demux9/1
  [v_Sa] -> Bus Creator2/1  "v(Sa)"
  Demux9/2 -> [v_Sc]
  [m_Sb] -> Demux8/1
  connections:
  D1/LConn1 -- S_a/LConn1 -- Diode Bridge/RConn1
  D2/RConn1 -- Diode Bridge/RConn2 -- S_a/RConn1
  Diode Bridge1/RConn2 -- S_b/RConn1 -- D4/RConn1
  Diode Bridge1/RConn1 -- S_b/LConn1 -- D3/LConn1
  Diode Bridge2/RConn2 -- S_c/RConn1 -- D6/RConn1
  Diode Bridge2/RConn1 -- S_c/LConn1 -- D5/LConn1
  Diode Bridge2/LConn1 -- C/RConn1
  Diode Bridge/LConn1 -- A/RConn1
  Diode Bridge1/LConn1 -- B/RConn1
  Diode Bridge/LConn2 -- DCn/RConn1 -- Diode Bridge2/LConn2 -- Diode Bridge1/LConn2
  D1/RConn1 -- DC+/RConn1 -- D5/RConn1 -- D3/RConn1
  D4/LConn1 -- D6/LConn1 -- DC-/RConn1 -- D2/LConn1
